simulink model "slezh_sost_u0"  (R2024a)
settings: Solver=FixedStepAuto  StartTime=0.0  StopTime=10.0  FixedStep=0.0001  RelTol=1e-3
values from neighbouring files (symbols this model uses):
  A = [11 -2 13; 6 -1 6; -6 -1 -8]    [comp_sost.m]    (also in meandr.m = [0 1; 0 0]; out.m; out_copy.m; rank_extended.m)
  Cz = [-2 3 -1]    [comp_sost.m]    (also in meandr.m = -C; out.m; out_copy.m = C; slezh_sost.m)
  Dz = 16/pi * [1 0 1/3 0 1/5 0]    [meandr.m]    (also in out.m = [3 4 2 -3]; out_copy.m = D; slezh_sost.m = [3 4 2 -3])
  G = [35 56 22 -42; -11 -17 -7 12; -6 -10 -5 10; 11 18 6 -13]    [comp_sost.m]    (also in meandr.m = [0 1 0 0 0 0; -1 0 0 0 0 0; 0 0 0 3 0 0; 0 0 -3 0 0 0; 0 0 0; out.m; out_copy.m; rank_extended.m)
settings Model: Creator=ventus  LastModifiedBy=ventus

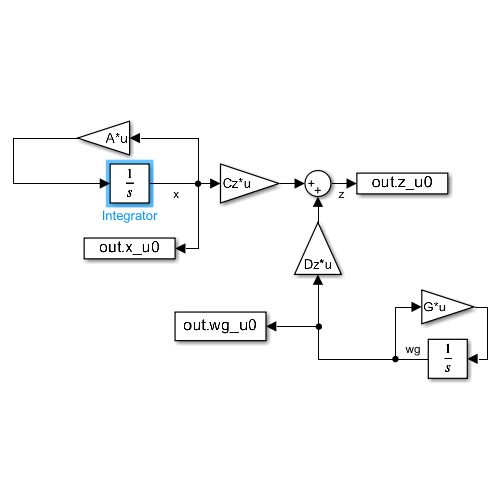
[thumbnail: Simulink's stored preview of the top-level diagram]
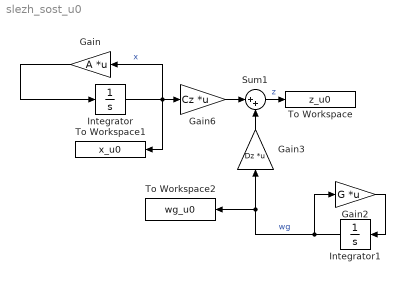
== system slezh_sost_u0 ==
  Gain : Gain  Gain=A  Multiplication=Matrix(K*u)
  Gain2 : Gain  Gain=G  Multiplication=Matrix(K*u)
  Gain3 : Gain  Gain=Dz  Multiplication=Matrix(K*u)
  Gain6 : Gain  Gain=Cz  Multiplication=Matrix(K*u)
  Integrator : Integrator  InitialCondition=[1; 1; 1]
  Integrator1 : Integrator  InitialCondition=[1; 1; 1; 1]
  Sum1 : Sum  Inputs=|++
  To Workspace : ToWorkspace  VariableName=z_u0  SaveFormat=Timeseries  SampleTime=-1
  To Workspace1 : ToWorkspace  VariableName=x_u0  SaveFormat=Timeseries  SampleTime=-1
  To Workspace2 : ToWorkspace  VariableName=wg_u0  SaveFormat=Timeseries  SampleTime=-1
  wires:
  Gain6/1 -> Sum1/1
  Sum1/1 -> To Workspace/1  "z"
  Gain2/1 -> Integrator1/1
  Integrator/1 -> Gain6/1, Gain/1, To Workspace1/1  "x"
  Gain3/1 -> Sum1/2
  Integrator1/1 -> Gain2/1, To Workspace2/1, Gain3/1  "wg"
  Gain/1 -> Integrator/1
